simulink model "problem5"  (R2020b)
settings: Solver=VariableStepAuto  StartTime=0.0  StopTime=10.0  RelTol=1e-3
undefined symbols (not defined in the file): C, R
settings Model: Creator=admin  LastModifiedBy=admin

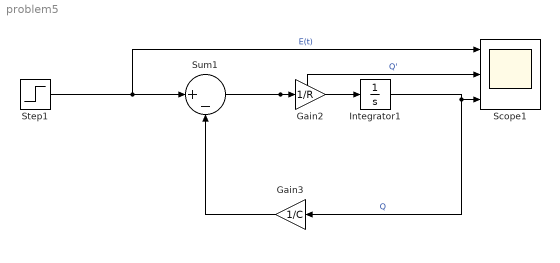
== system problem5 ==
  Gain2 : Gain  Gain=1/R
  Gain3 : Gain  Gain=1/C
  Integrator1 : Integrator
  Scope1 : Scope  NumInputPorts=3
  Step1 : Step  SampleTime=0
  Sum1 : Sum  Inputs=|+-
  wires:
  Step1/1 -> Scope1/1, Sum1/1  "E(t)"
  Gain3/1 -> Sum1/2
  Gain2/1 -> Integrator1/1
  Integrator1/1 -> Gain3/1, Scope1/3  "Q"
  Sum1/1 -> Scope1/2, Gain2/1  "Q'"
